simulink model "motor_wOpAmp"  (R2019b)
settings: Solver=ode45  StartTime=0.0  StopTime=10  MaxStep=1e-05  MinStep=1e-08  RelTol=1e-08  AbsTol=1e-08  EnableMultiTasking=on
PreLoadFcn:
  | MotorParam
InitFcn:
  | MotorParam
values from neighbouring files (symbols this model uses):
  A0 = 7.452e05    (= 745200)    [MotorParam.m]
  A1 = 0    [MotorParam.m]
  B0 = 3.134e05    (= 313400)    [MotorParam.m]
  B1 = 1    [MotorParam.m]
  B2 = 0    [MotorParam.m]
  Kb = 10.95103*10^-3    (= 0.01095103)    [MotorParam.m]
  Km = 10.9*10^-3    (= 0.0109)    [MotorParam.m]
  L = 0.227*10^-3    (= 0.000227)    [MotorParam.m]
  R = 5.31    [MotorParam.m]
settings Model: Creator=Leo  LastModifiedBy=debby
settings SolverCC: ZeroCrossAlgorithm=Adaptive
settings DataIOCC: SaveFormat=Array  SignalLoggingSaveFormat=ModelDataLogs  ReturnWorkspaceOutputs=off
settings OptimizationCC: ExpressionDepthLimit=2147483647  InitFltsAndDblsToZero=on  LifeSpan=inf
settings DebuggingCC: UnderspecifiedInitializationDetection=Classic  MergeDetectMultiDrivingBlocksExec=none  FcnCallInpInsideContextMsg=warning  StateNameClashWarn=warning  SFUnexpectedBacktrackingDiag=warning  SFNoUnconditionalDefaultTransitionDiag=warning  SFExecutionAtInitializationDiag=none  ArithmeticOperatorsInVariantConditions=warning
settings HardwareCC: ProdBitPerPointer=32  ProdBitPerSizeT=32  ProdBitPerPtrDiffT=32  ProdLargestAtomicFloat=None  ProdIntDivRoundTo=Undefined  ProdEndianess=Unspecified  ProdWordSize=32  ProdHWDeviceType=32-bit Generic
settings ModelReferenceCC: PropagateSignalLabelsOutOfModel=off
settings SFSimCC: SimUseLocalCustomCode=off  CustomCodeUndefinedFunction=UseInterfaceOnly
settings RTWCC: RTWUseLocalCustomCode=off
settings CodeAppCC: StateflowObjectComments=on
settings GRTTargetCC: TargetLangStandard=C89/C90 (ANSI)  GeneratePreprocessorConditionals=Disable all  CombineOutputUpdateFcns=off  GRTInterface=on
settings ConfigComp: CovMetricSettings=dw  CovHtmlReporting=on  CovSaveCumulativeToWorkspaceVar=on  CovSaveSingleToWorkspaceVar=on  CovExternalEMLEnable=off  CovSFcnEnable=off

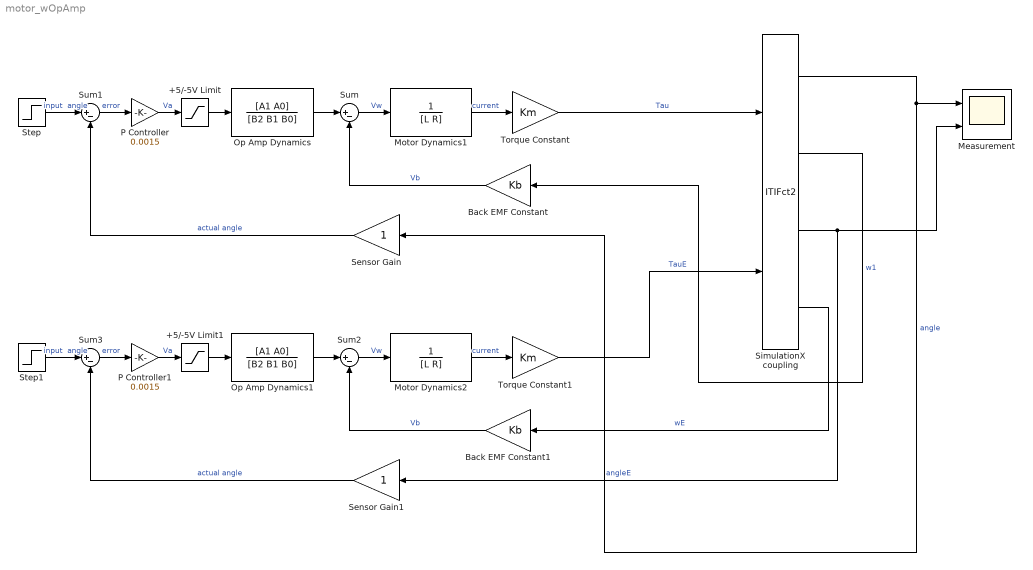
== system motor_wOpAmp ==
  +5/-5V Limit : Saturate  UpperLimit=5  LowerLimit=-5
  +5/-5V Limit1 : Saturate  UpperLimit=5  LowerLimit=-5
  Back EMF Constant : Gain  Gain=Kb
  Back EMF Constant1 : Gain  Gain=Kb
  Measurement : Scope  NumInputPorts=2
  Motor Dynamics1 : TransferFcn  Denominator=[L R]
  Motor Dynamics2 : TransferFcn  Denominator=[L R]
  Op Amp Dynamics : TransferFcn  Numerator=[A1 A0]  Denominator=[B2 B1 B0]
  Op Amp Dynamics1 : TransferFcn  Numerator=[A1 A0]  Denominator=[B2 B1 B0]
  P Controller : Gain  Gain=0.0015
  P Controller1 : Gain  Gain=0.0015
  Sensor Gain : Gain
  Sensor Gain1 : Gain
  SimulationX coupling : S-Function  FunctionName=ITIFct2  Parameters=ip, port, ts, nIn, nOut  SFunctionDeploymentMode=off  EnableBusSupport=off  mask{ip='localhost', port=1025, ts=0.001, nIn=2, nOut=4}
      mask prompts: ip "Address: ip"; port "Port Number: port [-]"; ts "Communication Step Size: ts [s]"; nIn "Input Vector Dimension (to SimulationX): nIn [-]"; nOut "Output Vector Dimension (from SimulationX): nOut [-]"
      mask help: Coupling Element
  Step : Step  Time=0.01  After=pi/2  SampleTime=0
  Step1 : Step  Time=0.01  After=pi/2  SampleTime=0
  Sum{,1..3} (4 alike) : Sum  Inputs=|+-
  Torque Constant : Gain  Gain=Km
  Torque Constant1 : Gain  Gain=Km
  wires:
  Sum/1 -> Motor Dynamics1/1  "Vw"
  Motor Dynamics1/1 -> Torque Constant/1  "current"
  Torque Constant/1 -> SimulationX coupling/1  "Tau"
  Back EMF Constant/1 -> Sum/2  "Vb"
  Op Amp Dynamics/1 -> Sum/1
  P Controller/1 -> +5/-5V Limit/1  "Va"
  +5/-5V Limit/1 -> Op Amp Dynamics/1
  Sum1/1 -> P Controller/1  "error"
  Step/1 -> Sum1/1  "input  angle"
  Sensor Gain/1 -> Sum1/2  "actual angle"
  Sum3/1 -> P Controller1/1  "error"
  Sensor Gain1/1 -> Sum3/2  "actual angle"
  P Controller1/1 -> +5/-5V Limit1/1  "Va"
  +5/-5V Limit1/1 -> Op Amp Dynamics1/1
  Back EMF Constant1/1 -> Sum2/2  "Vb"
  Sum2/1 -> Motor Dynamics2/1  "Vw"
  Motor Dynamics2/1 -> Torque Constant1/1  "current"
  Step1/1 -> Sum3/1  "input  angle"
  Op Amp Dynamics1/1 -> Sum2/1
  Torque Constant1/1 -> SimulationX coupling/2  "TauE"
  SimulationX coupling/1 -> Measurement/1, Sensor Gain/1  "angle"
  SimulationX coupling/2 -> Back EMF Constant/1  "w1"
  SimulationX coupling/3 -> Sensor Gain1/1, Measurement/2  "angleE"
  SimulationX coupling/4 -> Back EMF Constant1/1  "wE"
